simulink model "SteeringSimulation"  (R2020a)
settings: Solver=VariableStepAuto  StartTime=0.0  StopTime=50  RelTol=1e-3
libraries: simulink x1
settings Model: Creator=robot  LastModifiedBy=robot

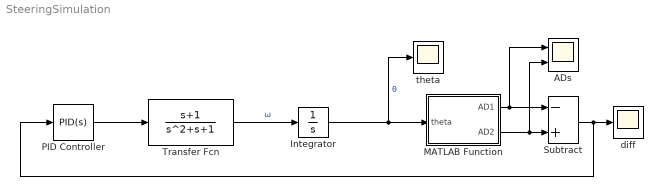
== system SteeringSimulation ==
  ADs : Scope  NumInputPorts=2
  Integrator : Integrator  InitialCondition=-1
  MATLAB Function : MATLAB Function  TreatAsAtomicUnit=on
  PID Controller : simulink/Continuous/PID Controller  Controller=PID  Form=Parallel  TimeDomain=Continuous-time  UseExternalTs=off  SampleTime=-1  IntegratorMethod=Forward Euler  FilterMethod=Forward Euler  ControllerParametersSource=internal  P=15.8218699709721  I=2.26814196058309  D=24.5225913069498  UseFilter=on  N=2808.2266335669  TunerSelectOption=Transfer Function Based (PID Tuner App)  InitialConditionSource=internal  InitialConditionForIntegrator=0  InitialConditionForFilter=0  DifferentiatorICPrevScaledInput=0  ExternalReset=none  TrackingMode=off  Kt=1  LimitOutput=off  UpperSaturationLimit=inf  LowerSaturationLimit=-inf  LinearizeAsGain=on  AntiWindupMode=none  Kb=1  POutMin=[]  POutMax=[]  IOutMin=[]  IOutMax=[]  DOutMin=[]  DOutMax=[]  NOutMin=[]  NOutMax=[]  SumOutMin=[]  SumOutMax=[]  SaturationOutMin=[]  SaturationOutMax=[]  PParamMin=[]  PParamMax=[]  IParamMin=[]  IParamMax=[]  DParamMin=[]  DParamMax=[]  NParamMin=[]  NParamMax=[]  KbParamMin=[]  KbParamMax=[]  KtParamMin=[]  KtParamMax=[]  KbOutMin=[]  KbOutMax=[]  KtOutMin=[]  KtOutMax=[]  IntegratorOutMin=[]  IntegratorOutMax=[]  FilterOutMin=[]  FilterOutMax=[]  SumI1OutMin=[]  SumI1OutMax=[]  SumI2OutMin=[]  SumI2OutMax=[]  SumI3OutMin=[]  SumI3OutMax=[]  SumI4OutMin=[]  SumI4OutMax=[]  SumDOutMin=[]  SumDOutMax=[]  DifferentiatorOutMin=[]  DifferentiatorOutMax=[]  FilterDiffOutCoefMin=[]  FilterDiffOutCoefMax=[]  ReciprocalOutMin=[]  ReciprocalOutMax=[]  SumDenOutMin=[]  SumDenOutMax=[]  SumNumOutMin=[]  SumNumOutMax=[]  DivideOutMin=[]  DivideOutMax=[]  UdiffTsProdOutMin=[]  UdiffTsProdOutMax=[]  NTsProdOutMin=[]  NTsProdOutMax=[]  UintegralTsProdOutMin=[]  UintegralTsProdOutMax=[]  UngainTsProdOutMin=[]  UngainTsProdOutMax=[]  IntegratorContinuousStateAttributes=''  IntegratorStateMustResolveToSignalObject=off  IntegratorRTWStateStorageClass=Auto  FilterContinuousStateAttributes=''  FilterStateMustResolveToSignalObject=off  FilterRTWStateStorageClass=Auto  ParallelPVariant=InternalParameters  IdealPVariant=Disabled  IVariant=InternalParameters  DVariant=InternalParameters  IntegratorVariant=Continuous  SatVariant=Disabled  AWVariant=Passthrough  PCopyVariant=Disabled  TRVariant=Disabled  FdbkBlocksVariant=Forward  IdealPFdbkVariant=Disabled  SatFdbkVariant=Disabled  DerivativeFilterVariant=ContFilter  NVariant=InternalParameters  NCopyVariant=Disabled  FilterICVariant=InternalICsFilter  IntegratorICVariant=InternalICs  ExternalResetVariant=Disabled  TRSumVariant=Passthrough  SumFdbkVariant=Disabled  SumVariant=Sum_PID  TsampFilterVariant=InternalTs  TsampNgainVariant=Passthrough  TsampIntegralVariant=Passthrough
  Subtract : Sum  Inputs=-+
  Transfer Fcn : TransferFcn  Numerator=[1 1]  Denominator=[1 1 1]
  diff : Scope
  theta : Scope
  wires:
  Transfer Fcn/1 -> Integrator/1  "ω"
  Integrator/1 -> theta/1, MATLAB Function/1(theta)  "θ"
  MATLAB Function/1(AD1) -> ADs/1, Subtract/1
  MATLAB Function/2(AD2) -> ADs/2, Subtract/2
  Subtract/1 -> PID Controller/1, diff/1
  PID Controller/1 -> Transfer Fcn/1

== matlab function SteeringSimulation/MATLAB Function ==
  data: theta input; AD1 output; AD2 output
function [AD1, AD2] = fcn(theta)
    % 左右のAD値はθ = 0付近では線形に変動するとしている。このAD値を実験データから求めた
    % 近似解の方程式に置き換えればPIDチューニングが可能かも？
    % また、ステアリングの伝達関数（または状態方程式）は無限に回転できる実験台に取り付けて
    % 実験してシステムどうすれば良いかも？

    F_ad1 = theta;
    F_ad2 = -theta;
    
    ad1 = 0;
    ad2 = 0;
    if theta > 0
        ad1 = F_ad1;
    elseif theta <= 0
        ad1 = 0; 
    end
    
    if theta > 0
        ad2 = 0;
    elseif theta <= 0
        ad2 = F_ad2; 
    end

    AD1 = ad1;
    AD2 = ad2;
end
